simulink model "Lab2_single_loop_controller_student"  (R2024b)
settings: Solver=FixedStepAuto  StartTime=0.0  StopTime=10  FixedStep=0.001  MaxStep=0.01  RelTol=1e-3
values from neighbouring files (symbols this model uses):
  g = 9.81    [Lab2_params_student.m]
  J = 2.20e-5 + mp*L^2    (= 0.000522)    [Lab2_params_student.m]
  ke = 0.057961    [Lab2_params_student.m]
  kt = 0.05630    (= 0.0563)    [Lab2_params_student.m]
  L = 0.1    [Lab2_params_student.m]
  Lm = 2.996e-3    (= 0.002996)    [Lab2_params_student.m]
  mp = 0.05    [Lab2_params_student.m]
  R = 2.556    [Lab2_params_student.m]
undefined symbols (not defined in the file or in its folder): X, Y, Z
libraries: sm_lib x14, nesl_utility x4
(part 1 of 2)
settings Model: Creator=User  LastModifiedBy=acer
settings RTWCC: GPUComputeCapability=3.5

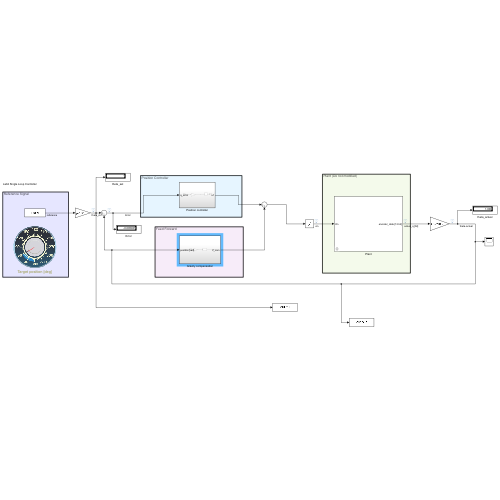
[thumbnail: Simulink's stored preview of the top-level diagram]
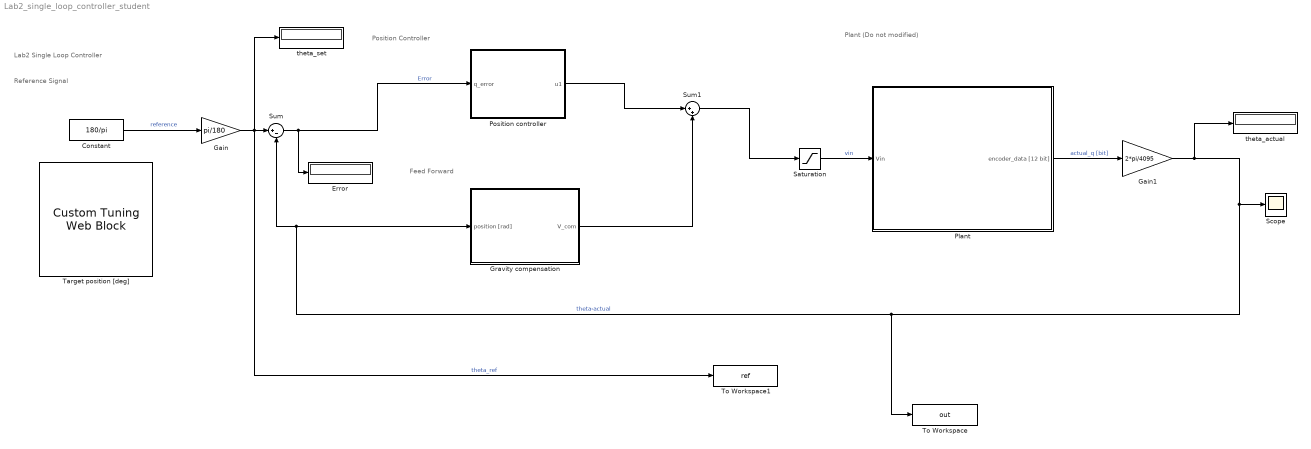
== system Lab2_single_loop_controller_student ==
  note: Lab2 Single Loop Controller
  note: Plant (Do not modified)
  note: Feed Forward
  note: Position Controller
  note: Reference Signal
  Constant : Constant  Value=180/pi  SampleTime=-1
  Error : Display
  Gain : Gain  Gain=pi/180
  Gain1 : Gain  Gain=2*pi/4095
  Gravity compensation : Subsystem
  Plant : Subsystem  mask{init_q=0}
      mask prompts: init_q "Initial angle of pendulum [deg]"
  Position controller : Subsystem
  Saturation : Saturate  UpperLimit=12  LowerLimit=-12
  Scope : Scope
  Sum : Sum  Inputs=|+-
  Sum1 : Sum  Inputs=|++
  Target position [deg] : CustomTuningWebBlock  LabelPosition=Hide  ShowInitialText=on  Configuration="{\"components\":[{\"name\":\"CircularScaleComponent\",\"settings\":{\"bounds\":{\"max\":360,\"min\":0,\"tickInterval\":30},\"direction\":\"cw\",\"flipLimits\":0,\"innerRadius\":0.6636618227670849,\"internalTickHeightScaleFactor\":1,\"labelColor\":[255,255,200],\"labelFont\":{\"font\":\"Arial\",\"fontSize\":12},\"labelRadius\":0.79,\"labelTransparency\":1,\"minorTickHeightScaleFactor\":0.2,\"needleImage\":{\"size\":[150,150],\"src\":\"data:image\\/svg+xml;base64,PD94bWwgdmVyc2lvbj0iMS4wIiBlbmNvZGluZz0idXRmLTgiPz4NCjwhLS0gR2VuZXJhdG9yOiBBZG9iZSBJbGx1c3RyYXRvciAyNS4yLjMsIFNWRyBFeHBvcnQgUGx1Zy1JbiAuIFNWRyBWZXJzaW9uOiA2LjAwIEJ1aWxkIDApICAtLT4NCjxzdmcgdmVyc2lvbj0iMS4xIiBpZD0iTGF5ZXJfMSIgeG1sbnM9Imh0dHA6Ly93d3cudzMub3JnLzIwMDAvc3ZnIiB4bWxuczp4bGluaz0iaHR0cDovL3d3dy53My5vcmcvMTk5OS94bGluayIgeD0iMHB4IiB5PSIwcHgiDQoJIHZpZXdCb3g9IjAgMCAxNTIgMTUyIiBzdHlsZT0iZW5hYmxl ...(+37472 chars)\"},\"needleOffset\":[0,0],\"needleOrientation\":-45,\"needleRotation\":90,\"needleSize\":{\"height\":0.44,\"width\":0.44},\"outerRadius\":0.5053386200069245,\"position\":[0,0,1,1],\"referencePoint\":\"auto\",\"scaleAngle\":360,\"scaleAngleOffset\":90,\"scaleColors\":[],\"scaleColorsSize\":0.2,\"scaleDirection\":\"CW\",\"scalePosition\":[0,0,1,1],\"showLabels\":1,\"showMinorTicks\":1,\"showSpanLine\":true,\"showTicks\":1,\"tickColor\":[252,252,197],\"tickTransparency\":1,\"valueBarColor\":[0,114,189],\"valueBarPosition\":[0,0,1,1],\"valueBarSize\":0.2,\"valueBarTransparency\":1}},{\"name\":\"BackgroundImageComponent\",\"settings\":{\"image\":{\"size\":[385,373],\"src\":\"data:image\\/svg+xml;base64,PD94bWwgdmVyc2lvbj0iMS4wIiBlbmNvZGluZz0idXRmLTgiPz4NCjwhLS0gR2VuZXJhdG9yOiBBZG9iZSBJbGx1c3RyYXRvciAyNS4wLjAsIFNWRyBFeHBvcnQgUGx1Zy1JbiAuIFNWRyBWZXJzaW9uOiA2LjAwIEJ1aWxkIDApICAtLT4NCjxzdmcgdmVyc2lvbj0iMS4xIg0KCSBpZD0iTGF5ZXJfMl8xXyIgeG1sbnM6Y2M9Imh0dHA6Ly9jcmVhdGl2ZWNvbW1vbnMub3JnL25zIyIgeG1sbnM6ZGM9Imh0dHA6Ly9wdXJsLm9yZy9kYy9lbGVtZW50cy8xLjEvIiB4bWxuczppbmtzY2FwZT0iaHR0cDovL3d3dy5pbmtzY2FwZS5vcmcv ...(+4184 chars)\",\"srcOrientation\":\"horizontal\"},\"position\":[0,0,1,1],\"scaleMode\":\"0\"}},{\"name\":\"ForegroundImageComponent\",\"settings\":{\"image\":{\"size\":[0,0],\"src\":\"default\",\"srcOrientation\":[]},\"isForeground\":1,\"position\":[0,0,1,1],\"scaleMode\":\"0\"}}],\"settings\":{\"BindingType\":\"param\",\"aspectRatio\":1,\"backgroundColor\":[0,0,0,\"1\"],\"backgroundOffset\":1,\"backgroundOpacity\":1,\"direction\":\"cw\",\"fixedAspectRatio\":\"off\",\"flipLimits\":0,\"foregroundColor\":[252,252,196],\"orientation\":\"horizontal\",\"showBackgroundColor\":false,\"value\":0,\"version\":\"R2023a\"},\"type\":\"CircularGauge\"}"
  To Workspace : ToWorkspace  VariableName=out  SaveFormat=Timeseries  SampleTime=-1
  To Workspace1 : ToWorkspace  VariableName=ref  SaveFormat=Timeseries  SampleTime=-1
  theta_actual : Display
  theta_set : Display
  wires:
  Saturation/1 -> Plant/1(Vin)  "vin"
  Constant/1 -> Gain/1  "reference"
  Gain/1 -> To Workspace1/1, theta_set/1, Sum/1  "theta_ref"
  Sum/1 -> Error/1, Position controller/1(q_error)  "Error"
  Plant/1(encoder_data [12 bit]) -> Gain1/1  "actual_q [bit]"
  Gain1/1 -> theta_actual/1, Scope/1, To Workspace/1, Sum/2, Gravity compensation/1(position [rad])  "theta-actual"
  Position controller/1(u1) -> Sum1/1
  Gravity compensation/1(V_com) -> Sum1/2
  Sum1/1 -> Saturation/1

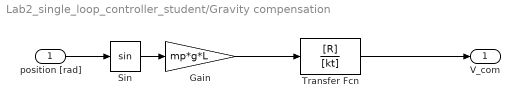
== system Lab2_single_loop_controller_student/Gravity compensation ==
  position [rad] : Inport
  Gain : Gain  Gain=mp*g*L
  Sin : Trigonometry
  Transfer Fcn : TransferFcn  Numerator=[R]  Denominator=[kt]
  V_com : Outport
  wires:
  position [rad]/1 -> Sin/1
  Sin/1 -> Gain/1
  Gain/1 -> Transfer Fcn/1
  Transfer Fcn/1 -> V_com/1

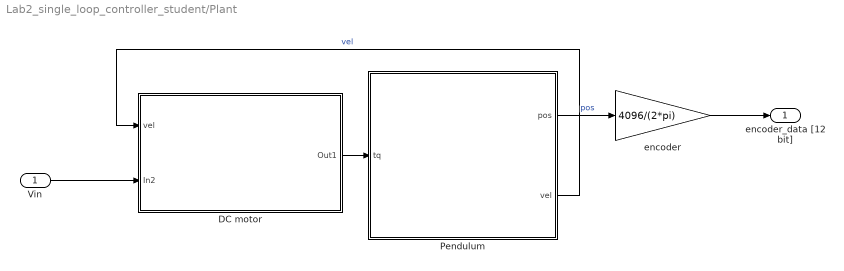
== system Lab2_single_loop_controller_student/Plant ==
  Vin : Inport
  DC motor : Subsystem
  Pendulum : Subsystem
      mask Display: image('simple_pendulum_brick.png'); % Use "Edit Image" on toolstrip to change.
  encoder : Gain  Gain=4096/(2*pi)
  encoder_data [12 bit] : Outport
  wires:
  Pendulum/1(pos) -> encoder/1  "pos"
  encoder/1 -> encoder_data [12 bit]/1
  Pendulum/2(vel) -> DC motor/1(vel)  "vel"
  Vin/1 -> DC motor/2(In2)
  DC motor/1(Out1) -> Pendulum/1(tq)

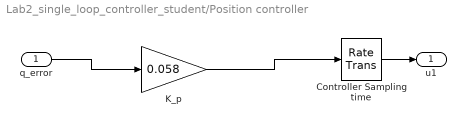
== system Lab2_single_loop_controller_student/Position controller ==
  q_error : Inport
  Controller Sampling time : RateTransition  OutPortSampleTime=0.001
  K_p : Gain  Gain=0.058
  u1 : Outport
  wires:
  Controller Sampling time/1 -> u1/1
  q_error/1 -> K_p/1
  K_p/1 -> Controller Sampling time/1

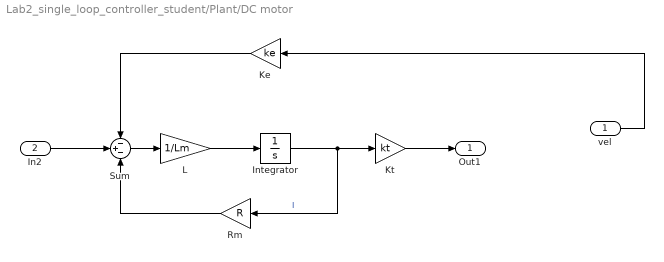
== system Lab2_single_loop_controller_student/Plant/DC motor ==
  vel : Inport
  In2 : Inport  Port=2
  Integrator : Integrator
  Ke : Gain  Gain=ke
  Kt : Gain  Gain=kt
  L : Gain  Gain=1/Lm
  Rm : Gain  Gain=R
  Sum : Sum  Inputs=-+-
  Out1 : Outport
  wires:
  vel/1 -> Ke/1
  In2/1 -> Sum/2
  Sum/1 -> L/1
  Rm/1 -> Sum/3
  Ke/1 -> Sum/1
  Kt/1 -> Out1/1
  Integrator/1 -> Kt/1, Rm/1  "I"
  L/1 -> Integrator/1
